simulink model "sltank2"  (Simulink 4.00)
settings: Solver=ode23  SolverMode=SingleTasking  StartTime=0  StopTime=10000  MaxStep=0.2  RelTol=1e-3  AbsTol=1e-6
PreLoadFcn:
  | tank2=readfis('tank2');
libraries: fuzblock x1, simulink_extras x1
settings Model: Creator=pascal  LastModifiedBy=pascal  SaveTime=off  SaveOutput=off  LimitDataPoints=off  ExtModeTrigMode=oneshot  ExtModeArmWhenConnect=off  BlockReductionOpt=off

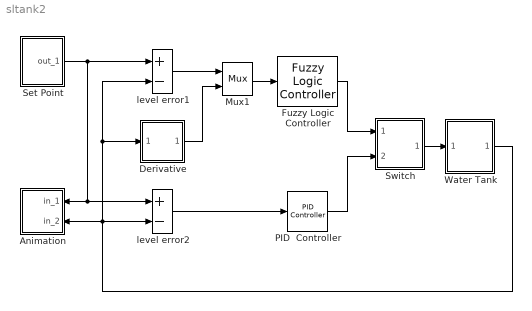
== system sltank2 ==
  Animation : Subsystem  Orientation=left
      settings: RTWFcnNameOpts=Auto  RTWFileNameOpts=Auto
  Derivative : Subsystem
      settings: RTWFcnNameOpts=Auto  RTWFileNameOpts=Auto
  Fuzzy Logic Controller : fuzblock/Fuzzy Logic  Controller  fis=tank2
  Mux1 : Mux  Inputs=2
      settings: DisplayOption=none
  PID  Controller : simulink_extras/Additional Linear/PID Controller  P=2  I=0  D=1
  Set Point : Subsystem
      settings: RTWFcnNameOpts=Auto  RTWFileNameOpts=Auto
  Switch : Subsystem
      settings: RTWFcnNameOpts=Auto  RTWFileNameOpts=Auto
  Water Tank : Subsystem
      settings: RTWFcnNameOpts=Auto  RTWFileNameOpts=Auto
  level error1 : Sum  Inputs=+-  SaturateOnIntegerOverflow=on
  level error2 : Sum  Inputs=+-  SaturateOnIntegerOverflow=on
  wires:
  Water Tank/1(out_1) -> Derivative/1(in_1), level error1/2, Animation/2(in_2), level error2/2
  level error2/1 -> PID  Controller/1
  Derivative/1(out_1) -> Mux1/2
  Set Point/1(out_1) -> level error2/1, Animation/1(in_1), level error1/1
  PID  Controller/1 -> Switch/2(in_2)
  Fuzzy Logic Controller/1 -> Switch/1(in_1)
  Switch/1(out_1) -> Water Tank/1(in_1)
  level error1/1 -> Mux1/1
  Mux1/1 -> Fuzzy Logic Controller/1

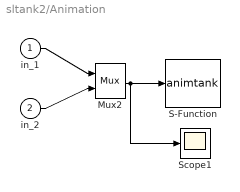
== system sltank2/Animation ==
  in_1 : Inport  Port=1
  in_2 : Inport  Port=2
  Mux2 : Mux  Inputs=2
      settings: DisplayOption=none
  S-Function : S-Function  FunctionName=animtank  Parameters=1  PortCounts=[]  SFunctionModules=''
  Scope1 : Scope
      settings: TickLabels=on  TimeRange=200.000000  YMin=-2.000000  YMax=2.000000  SaveToWorkspace=off  SaveName=ScopeData  DataFormat=Array  LimitDataPoints=on  MaxDataPoints=5000
  wires:
  in_2/1 -> Mux2/2
  in_1/1 -> Mux2/1
  Mux2/1 -> S-Function/1, Scope1/1

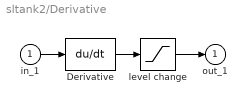
== system sltank2/Derivative ==
  in_1 : Inport  Port=1
  Derivative : Derivative
  level change : Saturate  UpperLimit=0.1  LowerLimit=-0.1  LinearizeAsGain=on
  out_1 : Outport  Port=1
  wires:
  in_1/1 -> Derivative/1
  level change/1 -> out_1/1
  Derivative/1 -> level change/1

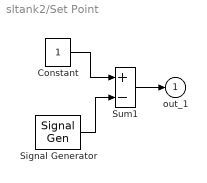
== system sltank2/Set Point ==
  Constant : Constant  Value=1
  Signal Generator : SignalGenerator  WaveForm=square  Amplitude=0.500000  Frequency=0.250000  Units=rad/sec
  Sum1 : Sum  Inputs=+-  SaturateOnIntegerOverflow=on
  out_1 : Outport  Port=1
  wires:
  Sum1/1 -> out_1/1
  Constant/1 -> Sum1/1
  Signal Generator/1 -> Sum1/2

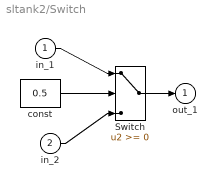
== system sltank2/Switch ==
  in_1 : Inport  Port=1
  in_2 : Inport  Port=2
  Switch : Switch  Threshold=0
  const : Constant  Value=0.5
  out_1 : Outport  Port=1
  wires:
  in_2/1 -> Switch/3
  Switch/1 -> out_1/1
  in_1/1 -> Switch/1
  const/1 -> Switch/2

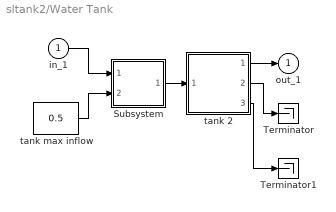
== system sltank2/Water Tank ==
  in_1 : Inport  Port=1
  Subsystem : Subsystem  mask(Valve){@1=0}
      mask prompts: @1 "Initial position [0=closed 1=open]:"
      mask help: Valve
      mask init:
      | InitialPosition = @1;
      settings: RTWFcnNameOpts=Auto  RTWFileNameOpts=Auto
      mask Display: disp('VALVE')
  Terminator : Terminator
  Terminator1 : Terminator
  tank 2 : Subsystem  mask(Water tank){@1=2, @2=1, @3=0.05, @4=0, @5=0.5}
      mask prompts: @1 "Height of tank (m):"; @2 "Bottom area (m^2):"; @3 "Out pipe crossection (m^2):"; @4 "Overflow sensor distance from top (m):"; @5 "Initial level height (m):"
      mask help: Cylindrical water tank with overflow signal
      mask init:
      | ht=@1;area=@2;outletArea=@3;overflowLimit=@4;initialHt=@5;
      settings: RTWFcnNameOpts=Auto  RTWFileNameOpts=Auto
      mask Display: disp('WATER\nTANK')
  tank max inflow : Constant  Value=0.5
  out_1 : Outport  Port=1
  wires:
  Subsystem/1(out flow) -> tank 2/1(flow in)
  tank max inflow/1 -> Subsystem/2(source flow)
  tank 2/1(water level) -> out_1/1
  in_1/1 -> Subsystem/1(control)
  tank 2/2(flow out) -> Terminator/1
  tank 2/3(overflow flag) -> Terminator1/1

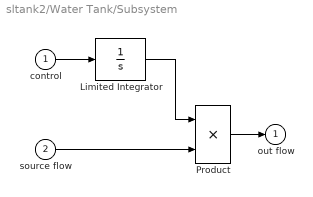
== system sltank2/Water Tank/Subsystem ==
  control : Inport  Port=1
  source flow : Inport  Port=2
  Limited Integrator : Integrator  ExternalReset=none  InitialConditionSource=internal  InitialCondition=InitialPosition  LimitOutput=on  UpperSaturationLimit=1  LowerSaturationLimit=0  ShowSaturationPort=off  ShowStatePort=off  AbsoluteTolerance=auto
  Product : Product  Inputs=2  Multiplication=Element-wise(.*)  SaturateOnIntegerOverflow=on
  out flow : Outport  Port=1
  wires:
  source flow/1 -> Product/2
  Product/1 -> out flow/1
  control/1 -> Limited Integrator/1
  Limited Integrator/1 -> Product/1

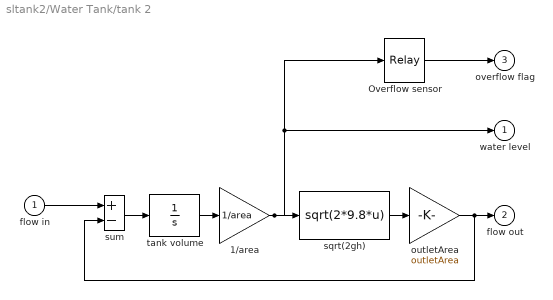
== system sltank2/Water Tank/tank 2 ==
  flow in : Inport  Port=1
  1/area : Gain  Gain=1/area  Multiplication=Element-wise(K.*u)  SaturateOnIntegerOverflow=on
  Overflow sensor : Relay  OnSwitchValue=ht - overflowLimit  OffSwitchValue=ht - overflowLimit  OnOutputValue=1  OffOutputValue=0
  outletArea : Gain  Gain=outletArea  Multiplication=Element-wise(K.*u)  SaturateOnIntegerOverflow=on
  sqrt(2gh) : Fcn  Expr=sqrt(2*9.8*u)
  sum : Sum  Inputs=+-  SaturateOnIntegerOverflow=on
  tank volume : Integrator  ExternalReset=none  InitialConditionSource=internal  InitialCondition=initialHt * area  LimitOutput=on  UpperSaturationLimit=ht * area  LowerSaturationLimit=0  ShowSaturationPort=off  ShowStatePort=off  AbsoluteTolerance=auto
  water level : Outport  Port=1
  flow out : Outport  Port=2
  overflow flag : Outport  Port=3
  wires:
  1/area/1 -> water level/1, Overflow sensor/1, sqrt(2gh)/1
  outletArea/1 -> sum/2, flow out/1
  sqrt(2gh)/1 -> outletArea/1
  tank volume/1 -> 1/area/1
  Overflow sensor/1 -> overflow flag/1
  flow in/1 -> sum/1
  sum/1 -> tank volume/1
